simulink model "v3_sim_lqr_sigma_r"  (R2023b)
settings: Solver=VariableStepAuto  StartTime=0.0  StopTime=100  RelTol=1e-10
values from neighbouring files (symbols this model uses):
  K_sigma = [K_sigma, K.']    [WP5.m]
  sigma = [0.01:0.02:2]    [WP5.m]
libraries: simulink x2
settings Model: Creator=kiraa  LastModifiedBy=kiraa

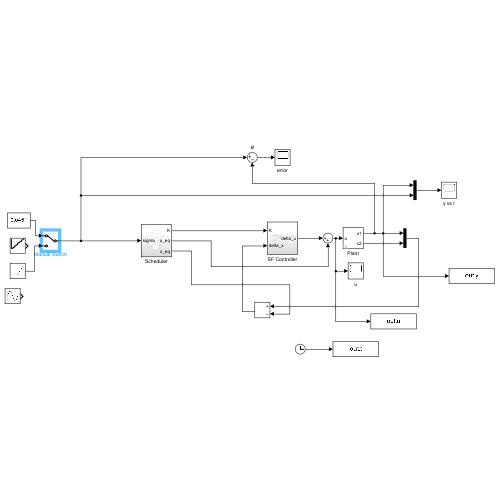
[thumbnail: Simulink's stored preview of the top-level diagram]
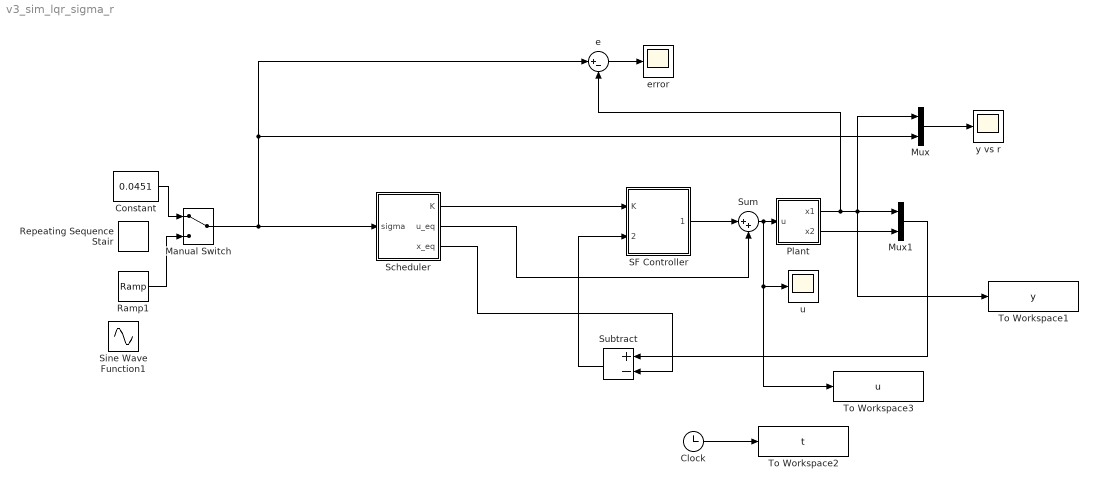
== system v3_sim_lqr_sigma_r ==
  Clock : Clock
  Constant : Constant  Value=0.0451
  Manual Switch : ManualSwitch
  Mux : Mux  Inputs=2
  Mux1 : Mux  Inputs=2
  Plant : Subsystem  mask{x1_0=0.1, x2_0=0}
      mask prompts: x1_0 "x1(0) [g/l]"; x2_0 "x2(0) [min^-1]"
  Ramp1 : simulink/Sources/Ramp  slope=-0.0005  start=0  InitialOutput=0.1
  Repeating Sequence Stair : simulink/Sources/Repeating Sequence Stair  OutValues=[0.1 0.2 0.3 0.4 0.5 0.6 0.7 0.8 0.9].'  tsamp=20  OutMin=[]  OutMax=[]  OutDataTypeStr=double  OutputDataTypeScalingMode=double  OutDataType=fixdt(0,8)  ConRadixGroup=Best Precision: Vector-wise  OutScaling=2^-12
  SF Controller : Subsystem
  Scheduler : Subsystem
  Sine Wave Function1 : Sin  Amplitude=0.02  Bias=0.05  Frequency=0.1  SampleTime=0
  Subtract : Sum  Inputs=+-
  Sum : Sum  Inputs=|++
  To Workspace1 : ToWorkspace  VariableName=y  SampleTime=-1
  To Workspace2 : ToWorkspace  VariableName=t  SampleTime=-1
  To Workspace3 : ToWorkspace  VariableName=u  SampleTime=-1
  e : Sum  Inputs=|+-
  error : Scope
  u : Scope
  y vs r : Scope
  wires:
  Plant/1(x1) -> To Workspace1/1, Mux1/1, Mux/1, e/2
  Mux/1 -> y vs r/1
  Constant/1 -> Manual Switch/1
  Manual Switch/1 -> Scheduler/1(sigma), Mux/2, e/1
  SF Controller/1(delta_u) -> Sum/1
  e/1 -> error/1
  Sum/1 -> u/1, To Workspace3/1, Plant/1(u)
  Subtract/1 -> SF Controller/2(delta_x)
  Plant/2(x2) -> Mux1/2
  Mux1/1 -> Subtract/1
  Scheduler/2(u_eq) -> Sum/2
  Scheduler/3(x_eq) -> Subtract/2
  Scheduler/1(K) -> SF Controller/1(K)
  Ramp1/1 -> Manual Switch/2
  Clock/1 -> To Workspace2/1

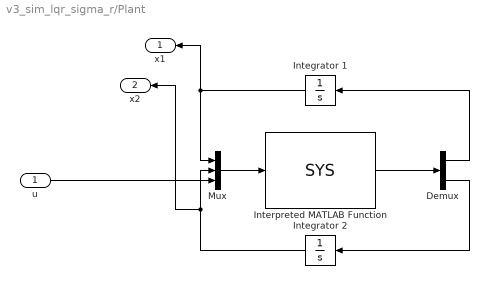
== system v3_sim_lqr_sigma_r/Plant ==
  u : Inport
  Demux : Demux  Outputs=2
  Integrator 1 : Integrator  InitialCondition=x1_0
  Integrator 2 : Integrator  InitialCondition=x2_0
  Interpreted MATLAB Function : MATLABFcn  MATLABFcn=SYS  OutputDimensions=2
  Mux : Mux  Inputs=3
  x1 : Outport
  x2 : Outport  Port=2
  wires:
  Integrator 1/1 -> x1/1, Mux/1
  Demux/1 -> Integrator 1/1
  Mux/1 -> Interpreted MATLAB Function/1
  Integrator 2/1 -> x2/1, Mux/2
  Interpreted MATLAB Function/1 -> Demux/1
  Demux/2 -> Integrator 2/1
  u/1 -> Mux/3

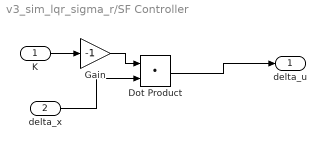
== system v3_sim_lqr_sigma_r/SF Controller ==
  K : Inport
  delta_x : Inport  Port=2
  Dot Product : DotProduct  OutDataTypeStr=Inherit: Inherit via internal rule
  Gain : Gain  Gain=-1
  delta_u : Outport
  wires:
  K/1 -> Gain/1
  Gain/1 -> Dot Product/1
  delta_x/1 -> Dot Product/2
  Dot Product/1 -> delta_u/1

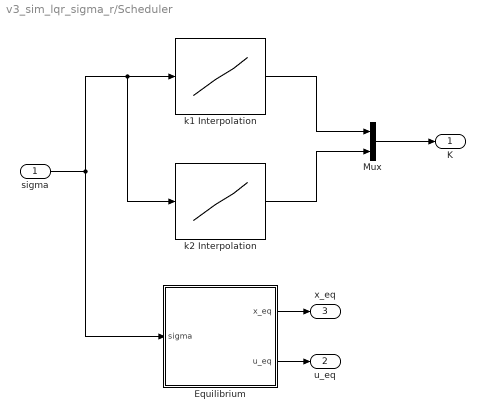
== system v3_sim_lqr_sigma_r/Scheduler ==
  sigma : Inport
  Equilibrium : MATLAB Function  TreatAsAtomicUnit=on
  Mux : Mux  Inputs=2
  k1 Interpolation : Lookup_n-D  NumberOfTableDimensions=1  BreakpointsForDimension1=sigma  Table=K_sigma(1,:)  InternalRulePriority=Speed  OutDataTypeStr=double  RndMeth=Simplest
  k2 Interpolation : Lookup_n-D  NumberOfTableDimensions=1  BreakpointsForDimension1=sigma  Table=K_sigma(2,:)  InternalRulePriority=Speed  OutDataTypeStr=double  RndMeth=Simplest
  K : Outport
  u_eq : Outport  Port=2
  x_eq : Outport  Port=3
  wires:
  Equilibrium/1(x_eq) -> x_eq/1
  Equilibrium/2(u_eq) -> u_eq/1
  sigma/1 -> k2 Interpolation/1, k1 Interpolation/1, Equilibrium/1(sigma)
  k1 Interpolation/1 -> Mux/1
  k2 Interpolation/1 -> Mux/2
  Mux/1 -> K/1

== matlab function v3_sim_lqr_sigma_r/Scheduler/Equilibrium ==
  data: sigma input; x_eq output; u_eq output
function [x_eq,u_eq] = compute_equilibrium(sigma)
    u_eq = -(399496308545527218176*sigma - 412936040625518808125)/(8736983277098762240000*sigma);
    x_eq = [sigma; -(1360087087465889792*sigma - 1319284474841913125)/(90071992547409920000*sigma)];
end
